simulink model "Simulation_empc_with_observer"  (Simulink 7.2)
settings: Solver=ode3  StartTime=0.0  StopTime=tend  FixedStep=TS  RelTol=accr
values from neighbouring files (symbols this model uses):
  A = A1    [Genetic_for_observer_matrices.m]    (also in Genetic_for_observer_matrices1.m; Ld.mat = [1  0.05; 0  1]; Ld1.mat = [1  0.05; 0  1]; Lx.mat = [1  0.05; 0  1])
  astinv = [0  0  1; 20  -10  0; 0  20  0]    [Ld.mat]    (also in Ld1.mat; Lx.mat; Lx1.mat; final_2integrator.m = inv([A-eye(2) B;C D]))
  B = [0.025 0.05]    [Ld.mat]    (also in Ld1.mat; Lx.mat; Lx1.mat; My_eMPC_Matrices_x.m = sysStruct.B)
  C = C1    [Genetic_for_observer_matrices.m]    (also in Genetic_for_observer_matrices1.m; Ld.mat = [1 0]; Ld1.mat = [1 0]; Lx.mat = [1 0])
  distAmp = 0.5    [Ld.mat]    (also in Ld1.mat; Lx.mat; Lx1.mat; final_2integrator.m)
  Ld = [p(1)]    [Constraint_for_observer_matrices.m]    (also in Ld.mat = -0.125285844408; Ld1.mat = -0.125285844408; Lx.mat = -0.125285844408; Lx1.mat = -0.125285844408)
  Ld1 = -0.609267812348    [Ld.mat]    (also in Ld1.mat; Lx.mat; Lx1.mat)
  Lx = [p(2);p(3)]    [Constraint_for_observer_matrices.m]    (also in Ld.mat = [-0.74280026683 1.0965708725]; Ld1.mat = [-0.74280026683 1.0965708725]; Lx.mat = [-0.74280026683 1.0965708725]; Lx1.mat = [-0.74280026683 1.0965708725])
  Lx1 = [-1.65921969337 -1.60852548001]    [Ld.mat]    (also in Ld1.mat; Lx.mat; Lx1.mat)
  state_dec = 3    [Ld.mat]    (also in Ld1.mat; Lx.mat; Lx1.mat; final_2integrator.m = 2)
  sysStruct =     [Ld.mat]    (also in Ld1.mat; Lx.mat; Lx1.mat)
  T = T1    [Genetic_for_observer_matrices.m]    (also in Genetic_for_observer_matrices1.m; Ld.mat = [1 1]; Ld1.mat = [1 1]; Lx.mat = [1 1])
  tdist = 4    [Ld.mat]    (also in Ld1.mat; Lx.mat; Lx1.mat; final_2integrator.m = 7.5)
  theta0 = 0    [Ld.mat]    (also in Ld1.mat; Lx.mat; Lx1.mat; final_2integrator.m)
  TS = 0.05    [Ld.mat]    (also in Ld1.mat; Lx.mat; Lx1.mat; final_2integrator.m)
  x0 = [-0.5 0.6]    [Ld.mat]    (also in Ld1.mat; Lx.mat; Lx1.mat; final_2integrator.m = [-0.5;0.6])
  yref = 0.5    [Ld.mat]    (also in Ld1.mat; Lx.mat; Lx1.mat; final_2integrator.m)
settings Model: Creator=MohammadAli  LastModifiedBy=MohammadAli

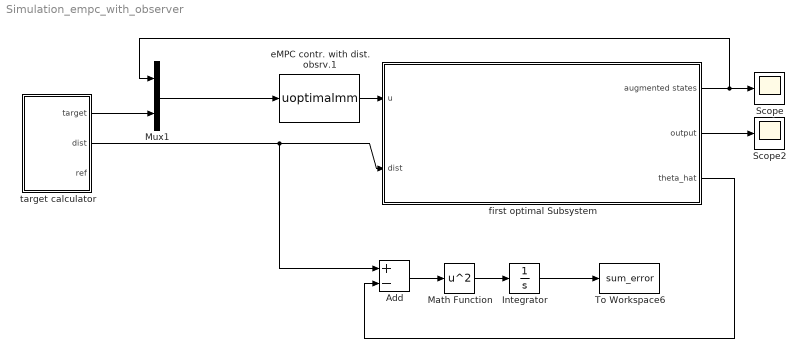
== system Simulation_empc_with_observer ==
  Add : Sum  Inputs=+-  OutDataType=sfix(16)  OutScaling=2^-10
  Integrator : Integrator
  Math Function : Math  Operator=square  OutDataType=sfix(16)  OutScaling=2^0  SaturateOnIntegerOverflow=on
  Mux1 : Mux  Inputs=2
  Scope : Scope
  Scope2 : Scope
      settings: SaveName=ScopeData4
  To Workspace6 : ToWorkspace  VariableName=sum_error  SampleTime=-1  SaveFormat=Structure With Time
  eMPC contr. with dist. obsrv.1 : MATLABFcn  MATLABFcn=uoptimalmm  Output1D=off  SampleTime=TS
  first optimal Subsystem : Subsystem
  target calculator : Subsystem
  wires:
  target calculator/1(target) -> Mux1/2
  first optimal Subsystem/1(augmented states) -> Mux1/1, Scope/1
  Mux1/1 -> eMPC contr. with dist. obsrv.1/1
  target calculator/2(dist) -> first optimal Subsystem/2(dist), Add/1
  eMPC contr. with dist. obsrv.1/1 -> first optimal Subsystem/1(u)
  first optimal Subsystem/2(output) -> Scope2/1
  Add/1 -> Math Function/1
  Math Function/1 -> Integrator/1
  Integrator/1 -> To Workspace6/1
  first optimal Subsystem/3(theta_hat) -> Add/2

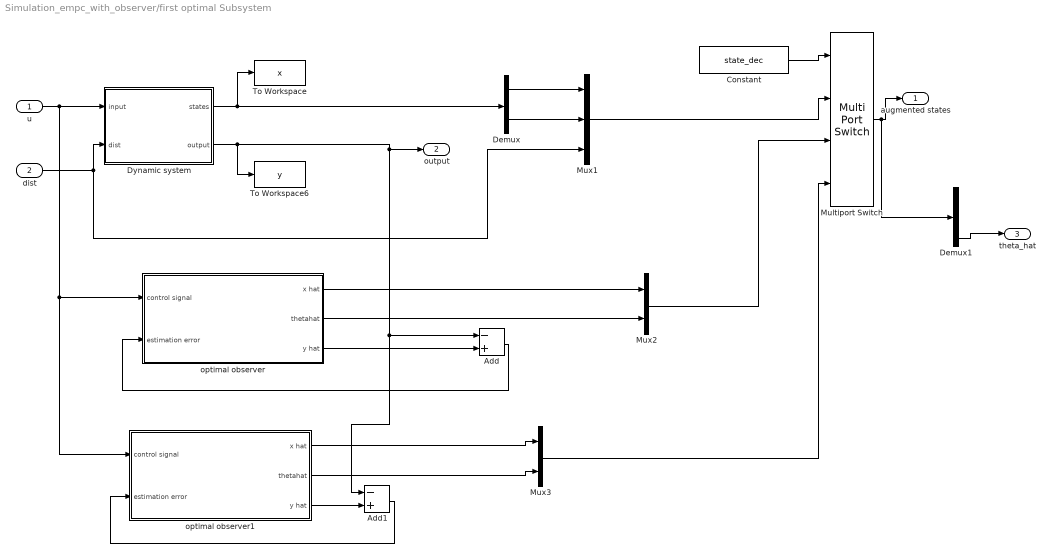
== system Simulation_empc_with_observer/first optimal Subsystem ==
  u : Inport
  dist : Inport  Port=2
  Add : Sum  Inputs=-+  OutDataType=sfix(16)  OutScaling=2^-10
  Add1 : Sum  Inputs=-+  OutDataType=sfix(16)  OutScaling=2^-10
  Constant : Constant  Value=state_dec  OutDataType=fixdt(1, 16)  OutScaling=2^0
  Demux : Demux  Outputs=2
  Demux1 : Demux  Outputs=3
  Dynamic system : Subsystem
  Multiport Switch : MultiPortSwitch  OutDataType=fixdt(1, 16)  OutScaling=2^0
  Mux1 : Mux  Inputs=3
  Mux2 : Mux  Inputs=2
  Mux3 : Mux  Inputs=2
  To Workspace : ToWorkspace  VariableName=x  SampleTime=-1  SaveFormat=Structure With Time
  To Workspace6 : ToWorkspace  VariableName=y  SampleTime=-1  SaveFormat=Structure With Time
  optimal observer : Subsystem
  optimal observer1 : Subsystem
  augmented states : Outport
  output : Outport  Port=2
  theta_hat : Outport  Port=3
  wires:
  Demux/1 -> Mux1/1
  Demux/2 -> Mux1/2
  Dynamic system/1(states) -> Demux/1, To Workspace/1
  optimal observer/3(y hat) -> Add/2
  Dynamic system/2(output) -> To Workspace6/1, Add1/1, Add/1, output/1
  Add/1 -> optimal observer/2(estimation error)
  optimal observer/1(x hat) -> Mux2/1
  optimal observer/2(thetahat) -> Mux2/2
  Mux1/1 -> Multiport Switch/2
  Mux2/1 -> Multiport Switch/3
  Constant/1 -> Multiport Switch/1
  dist/1 -> Dynamic system/2(dist), Mux1/3
  u/1 -> Dynamic system/1(input), optimal observer/1(control signal), optimal observer1/1(control signal)
  Multiport Switch/1 -> augmented states/1, Demux1/1
  optimal observer1/3(y hat) -> Add1/2
  Add1/1 -> optimal observer1/2(estimation error)
  optimal observer1/2(thetahat) -> Mux3/2
  optimal observer1/1(x hat) -> Mux3/1
  Mux3/1 -> Multiport Switch/4
  Demux1/3 -> theta_hat/1

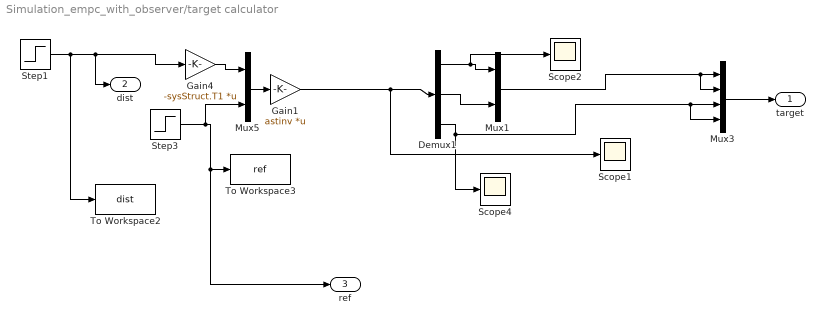
== system Simulation_empc_with_observer/target calculator ==
  Demux1 : Demux  Outputs=3
  Gain1 : Gain  Gain=astinv  Multiplication=Matrix(K*u)  ParameterDataType=sfix(16)  ParameterScaling=2^0  OutDataType=sfix(16)  OutScaling=2^0
  Gain4 : Gain  Gain=-sysStruct.T1  Multiplication=Matrix(K*u)  ParameterDataType=sfix(16)  ParameterScaling=2^0  OutDataType=sfix(16)  OutScaling=2^0
  Mux1 : Mux  Inputs=2
  Mux3 : Mux
  Mux5 : Mux  Inputs=2
  Scope1 : Scope
      settings: SaveName=ScopeData2
  Scope2 : Scope
      settings: SaveName=ScopeData3
  Scope4 : Scope
      settings: SaveName=ScopeData5
  Step1 : Step  Time=tdist  After=distAmp  SampleTime=0
  Step3 : Step  Time=0  After=yref  SampleTime=0
  To Workspace2 : ToWorkspace  VariableName=dist  SampleTime=-1  SaveFormat=Structure With Time
  To Workspace3 : ToWorkspace  VariableName=ref  SampleTime=-1  SaveFormat=Structure With Time
  target : Outport
  dist : Outport  Port=2
  ref : Outport  Port=3
  wires:
  Step3/1 -> Mux5/2, To Workspace3/1, ref/1
  Gain4/1 -> Mux5/1
  Mux5/1 -> Gain1/1
  Step1/1 -> Gain4/1, dist/1, To Workspace2/1
  Gain1/1 -> Demux1/1, Scope1/1
  Mux3/1 -> target/1
  Demux1/1 -> Mux1/1, Scope2/1
  Demux1/2 -> Mux1/2
  Mux1/1 -> Mux3/1, Mux3/2
  Demux1/3 -> Mux3/3, Mux3/4, Scope4/1

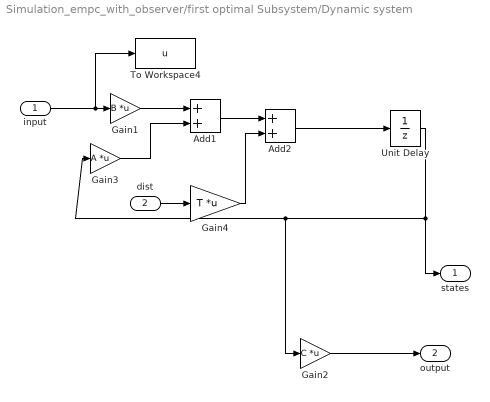
== system Simulation_empc_with_observer/first optimal Subsystem/Dynamic system ==
  input : Inport
  dist : Inport  Port=2
  Add1 : Sum  OutDataType=sfix(16)  OutScaling=2^-10
  Add2 : Sum  OutDataType=sfix(16)  OutScaling=2^-10
  Gain1 : Gain  Gain=B  Multiplication=Matrix(K*u)  ParameterDataType=sfix(16)  ParameterScaling=2^0  OutDataType=sfix(16)  OutScaling=2^0
  Gain2 : Gain  Gain=C  Multiplication=Matrix(K*u)  ParameterDataType=sfix(16)  ParameterScaling=2^0  OutDataType=sfix(16)  OutScaling=2^0
  Gain3 : Gain  Gain=A  Multiplication=Matrix(K*u)  ParameterDataType=sfix(16)  ParameterScaling=2^0  OutDataType=sfix(16)  OutScaling=2^0
  Gain4 : Gain  Gain=T  Multiplication=Matrix(K*u)  ParameterDataType=sfix(16)  ParameterScaling=2^0  OutDataType=sfix(16)  OutScaling=2^0
  To Workspace4 : ToWorkspace  VariableName=u  SampleTime=-1  SaveFormat=Structure With Time
  Unit Delay : UnitDelay  X0=x0  SampleTime=TS
  states : Outport
  output : Outport  Port=2
  wires:
  Gain3/1 -> Add1/2
  input/1 -> To Workspace4/1, Gain1/1
  Add1/1 -> Add2/1
  Unit Delay/1 -> Gain3/1, Gain2/1, states/1
  Add2/1 -> Unit Delay/1
  dist/1 -> Gain4/1
  Gain4/1 -> Add2/2
  Gain1/1 -> Add1/1
  Gain2/1 -> output/1

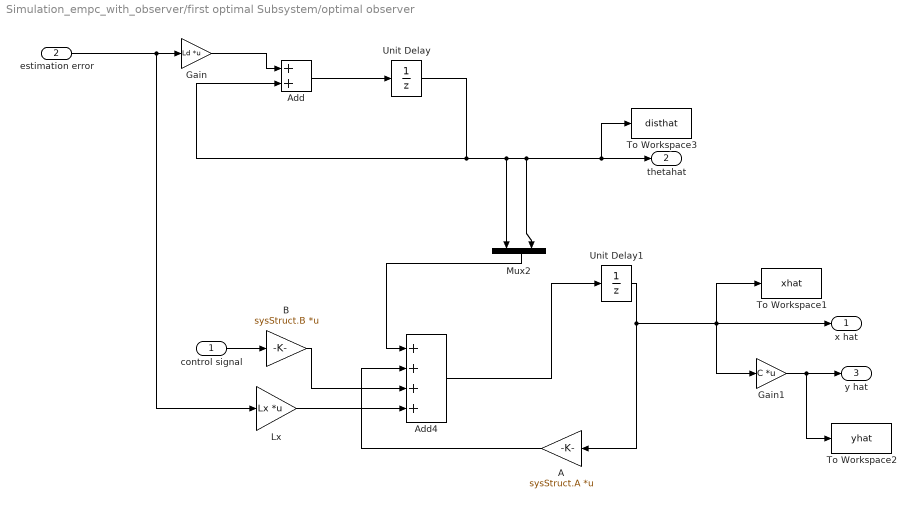
== system Simulation_empc_with_observer/first optimal Subsystem/optimal observer ==
  control signal : Inport
  estimation error : Inport  Port=2
  A : Gain  Orientation=left  Gain=sysStruct.A  Multiplication=Matrix(K*u)  ParameterDataType=sfix(16)  ParameterScaling=2^0  OutDataType=sfix(16)  OutScaling=2^0
  Add : Sum  OutDataType=sfix(16)  OutScaling=2^-10
  Add4 : Sum  Inputs=++++  OutDataType=sfix(16)  OutScaling=2^-10
  B : Gain  Gain=sysStruct.B  Multiplication=Matrix(K*u)  ParameterDataType=sfix(16)  ParameterScaling=2^0  OutDataType=sfix(16)  OutScaling=2^0
  Gain : Gain  Gain=Ld  Multiplication=Matrix(K*u)  ParameterDataType=sfix(16)  ParameterScaling=2^0  OutDataType=sfix(16)  OutScaling=2^0
  Gain1 : Gain  Gain=C  Multiplication=Matrix(K*u)  ParameterDataType=sfix(16)  ParameterScaling=2^0  OutDataType=sfix(16)  OutScaling=2^0
  Lx : Gain  Gain=Lx  Multiplication=Matrix(K*u)  ParameterDataType=sfix(16)  ParameterScaling=2^0  OutDataType=sfix(16)  OutScaling=2^0
  Mux2 : Mux  Orientation=down  Inputs=2
  To Workspace1 : ToWorkspace  VariableName=xhat  SampleTime=-1  SaveFormat=Structure With Time
  To Workspace2 : ToWorkspace  VariableName=yhat  SampleTime=-1  SaveFormat=Structure With Time
  To Workspace3 : ToWorkspace  VariableName=disthat  SampleTime=-1  SaveFormat=Structure With Time
  Unit Delay : UnitDelay  X0=theta0  SampleTime=TS
  Unit Delay1 : UnitDelay  X0=x0  SampleTime=TS
  x hat : Outport
  thetahat : Outport  Port=2
  y hat : Outport  Port=3
  wires:
  estimation error/1 -> Gain/1, Lx/1
  Gain/1 -> Add/1
  Add/1 -> Unit Delay/1
  Unit Delay/1 -> Add/2, Mux2/2, thetahat/1, To Workspace3/1, Mux2/1
  control signal/1 -> B/1
  Unit Delay1/1 -> A/1, x hat/1, Gain1/1, To Workspace1/1
  A/1 -> Add4/2
  Mux2/1 -> Add4/1
  B/1 -> Add4/3
  Lx/1 -> Add4/4
  Add4/1 -> Unit Delay1/1
  Gain1/1 -> y hat/1, To Workspace2/1

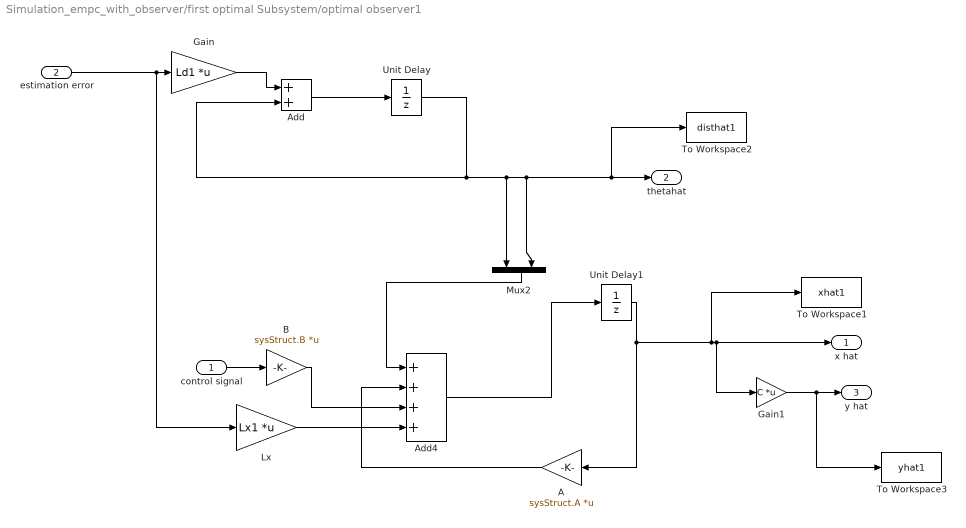
== system Simulation_empc_with_observer/first optimal Subsystem/optimal observer1 ==
  control signal : Inport
  estimation error : Inport  Port=2
  A : Gain  Orientation=left  Gain=sysStruct.A  Multiplication=Matrix(K*u)  ParameterDataType=sfix(16)  ParameterScaling=2^0  OutDataType=sfix(16)  OutScaling=2^0
  Add : Sum  OutDataType=sfix(16)  OutScaling=2^-10
  Add4 : Sum  Inputs=++++  OutDataType=sfix(16)  OutScaling=2^-10
  B : Gain  Gain=sysStruct.B  Multiplication=Matrix(K*u)  ParameterDataType=sfix(16)  ParameterScaling=2^0  OutDataType=sfix(16)  OutScaling=2^0
  Gain : Gain  Gain=Ld1  Multiplication=Matrix(K*u)  ParameterDataType=sfix(16)  ParameterScaling=2^0  OutDataType=sfix(16)  OutScaling=2^0
  Gain1 : Gain  Gain=C  Multiplication=Matrix(K*u)  ParameterDataType=sfix(16)  ParameterScaling=2^0  OutDataType=sfix(16)  OutScaling=2^0
  Lx : Gain  Gain=Lx1  Multiplication=Matrix(K*u)  ParameterDataType=sfix(16)  ParameterScaling=2^0  OutDataType=sfix(16)  OutScaling=2^0
  Mux2 : Mux  Orientation=down  Inputs=2
  To Workspace1 : ToWorkspace  VariableName=xhat1  SampleTime=-1  SaveFormat=Structure With Time
  To Workspace2 : ToWorkspace  VariableName=disthat1  SampleTime=-1  SaveFormat=Structure With Time
  To Workspace3 : ToWorkspace  VariableName=yhat1  SampleTime=-1  SaveFormat=Structure With Time
  Unit Delay : UnitDelay  X0=theta0  SampleTime=TS
  Unit Delay1 : UnitDelay  X0=x0  SampleTime=TS
  x hat : Outport
  thetahat : Outport  Port=2
  y hat : Outport  Port=3
  wires:
  Gain1/1 -> y hat/1, To Workspace3/1
  Add4/1 -> Unit Delay1/1
  Lx/1 -> Add4/4
  B/1 -> Add4/3
  Mux2/1 -> Add4/1
  A/1 -> Add4/2
  Unit Delay1/1 -> A/1, Gain1/1, x hat/1, To Workspace1/1
  control signal/1 -> B/1
  Unit Delay/1 -> Add/2, Mux2/1, Mux2/2, thetahat/1, To Workspace2/1
  Add/1 -> Unit Delay/1
  Gain/1 -> Add/1
  estimation error/1 -> Lx/1, Gain/1
